simulink model "Realistic_Model"  (R2019a)
settings: Solver=FixedStepAuto  StartTime=0.0  StopTime=200  FixedStep=dt  RelTol=1e-3
values from neighbouring files (symbols this model uses):
  phase_1 = 0    [initMonteCarlo.m]    (also in initRealModel.m; initTrapModel.m)
  phase_2 = 0.005    [initMonteCarlo.m]    (also in initRealModel.m = 0; initTrapModel.m)
  phase_3 = 0    [initRealModel.m]
  phase_4 = 0    [initRealModel.m]
  Q1 = 0.5*60*1000000000    (= 30000000000)    [initMonteCarlo.m]    (also in initRealModel.m = 2000; initTrapModel.m)
  Q2 = 0.5*60*1000000000    (= 30000000000)    [initMonteCarlo.m]    (also in initRealModel.m = 2000; initTrapModel.m)
  Q3 = 2000    [initRealModel.m]
  Q4 = 2000    [initRealModel.m]
  rate_1 = 0.01    [initMonteCarlo.m]    (also in initRealModel.m = 0.3; initTrapModel.m)
  rate_2 = 0.01    [initMonteCarlo.m]    (also in initRealModel.m = 0.3; initTrapModel.m)
  rate_3 = 0.3    [initRealModel.m]
  rate_4 = 0.3    [initRealModel.m]
  seed_1 = 0    [initMonteCarlo.m]    (also in initRealModel.m; initTrapModel.m)
  seed_2 = 1    [initMonteCarlo.m]    (also in initRealModel.m; initTrapModel.m)
  seed_3 = 2    [initRealModel.m]
  seed_4 = 3    [initRealModel.m]
libraries: simulink x8, SinglePipe_lib x7, Junction_Lib x3
settings Model: Creator=martin  LastModifiedBy=martin

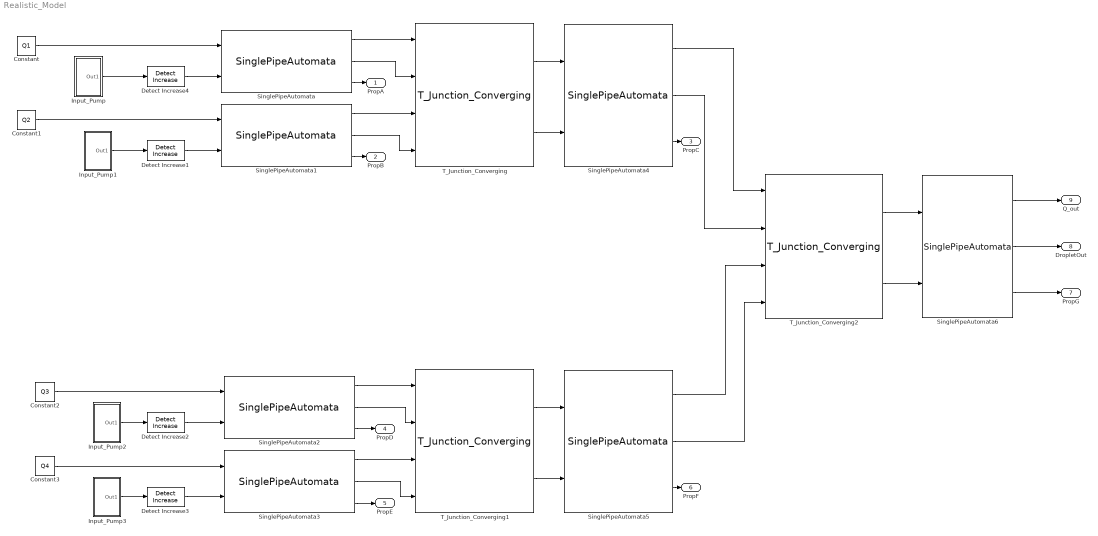
== system Realistic_Model ==
  Constant : Constant  Value=Q1
  Constant1 : Constant  Value=Q2
  Constant2 : Constant  Value=Q3
  Constant3 : Constant  Value=Q4
  Detect Increase{1..4} (4 alike) : simulink/Logic and Bit Operations/Detect Increase  vinit=0  OutDataTypeStr=boolean
  Input_Pump : Subsystem  mask{Period=rate_1, Seed=seed_1, PhaseDelay=phase_1}
      mask prompts: Period "droplet rate"; Seed "Simulink:blkprm_prompts:RandNumInitSeed"; PhaseDelay "Simulink:blkprm_prompts:PulseContPhaseDelay"
      mask TypeOptions Period:
      | Pulse
      | Generator/Period
      mask TypeOptions Seed:
      | Uniform Random
      | Number4/Seed
      mask TypeOptions PhaseDelay:
      | Pulse
      | Generator/PhaseDelay
      mask DialogControl Seed Prompt: Seed:
      mask DialogControl PhaseDelay Prompt: Phase delay (secs):
  Input_Pump1 : Subsystem  mask{Period=rate_2, Seed=seed_2, PhaseDelay=phase_2}
      mask prompts: Period "droplet rate"; Seed "Simulink:blkprm_prompts:RandNumInitSeed"; PhaseDelay "Simulink:blkprm_prompts:PulseContPhaseDelay"
      mask TypeOptions Period:
      | Pulse
      | Generator/Period
      mask TypeOptions Seed:
      | Uniform Random
      | Number4/Seed
      mask TypeOptions PhaseDelay:
      | Pulse
      | Generator/PhaseDelay
      mask DialogControl Seed Prompt: Seed:
      mask DialogControl PhaseDelay Prompt: Phase delay (secs):
  Input_Pump2 : Subsystem  mask{Period=rate_3, Seed=seed_3, PhaseDelay=phase_3}
      mask prompts: Period "droplet rate"; Seed "Simulink:blkprm_prompts:RandNumInitSeed"; PhaseDelay "Simulink:blkprm_prompts:PulseContPhaseDelay"
      mask TypeOptions Period:
      | Pulse
      | Generator/Period
      mask TypeOptions Seed:
      | Uniform Random
      | Number4/Seed
      mask TypeOptions PhaseDelay:
      | Pulse
      | Generator/PhaseDelay
      mask DialogControl Seed Prompt: Seed:
      mask DialogControl PhaseDelay Prompt: Phase delay (secs):
  Input_Pump3 : Subsystem  mask{Period=rate_4, Seed=seed_4, PhaseDelay=phase_4}
      mask prompts: Period "droplet rate"; Seed "Simulink:blkprm_prompts:RandNumInitSeed"; PhaseDelay "Simulink:blkprm_prompts:PulseContPhaseDelay"
      mask TypeOptions Period:
      | Pulse
      | Generator/Period
      mask TypeOptions Seed:
      | Uniform Random
      | Number4/Seed
      mask TypeOptions PhaseDelay:
      | Pulse
      | Generator/PhaseDelay
      mask DialogControl Seed Prompt: Seed:
      mask DialogControl PhaseDelay Prompt: Phase delay (secs):
  SinglePipeAutomata : SinglePipe_lib/SinglePipeAutomata  width=W.A  length=L.A  height=H.A  dt=dt
  SinglePipeAutomata1 : SinglePipe_lib/SinglePipeAutomata  width=W.B  length=L.B  height=H.B  dt=dt
  SinglePipeAutomata2 : SinglePipe_lib/SinglePipeAutomata  width=W.D  length=L.D  height=H.D  dt=dt
  SinglePipeAutomata3 : SinglePipe_lib/SinglePipeAutomata  width=W.E  length=L.E  height=H.E  dt=dt
  SinglePipeAutomata4 : SinglePipe_lib/SinglePipeAutomata  width=W.C  length=L.C  height=H.C  dt=dt
  SinglePipeAutomata5 : SinglePipe_lib/SinglePipeAutomata  width=W.F  length=L.F  height=H.F  dt=dt
  SinglePipeAutomata6 : SinglePipe_lib/SinglePipeAutomata  width=W.G  length=L.G  height=H.G  dt=dt
  T_Junction_Converging : Junction_Lib/T_Junction_Converging  SystemSampleTime=-1
  T_Junction_Converging1 : Junction_Lib/T_Junction_Converging  SystemSampleTime=-1
  T_Junction_Converging2 : Junction_Lib/T_Junction_Converging  SystemSampleTime=-1
  PropA : Outport
  PropB : Outport  Port=2
  PropC : Outport  Port=3
  PropD : Outport  Port=4
  PropE : Outport  Port=5
  PropF : Outport  Port=6
  PropG : Outport  Port=7
  DropletOut : Outport  Port=8
  Q_out : Outport  Port=9
  wires:
  T_Junction_Converging2/1 -> SinglePipeAutomata6/1
  T_Junction_Converging2/2 -> SinglePipeAutomata6/2
  SinglePipeAutomata4/1 -> T_Junction_Converging2/1
  SinglePipeAutomata4/2 -> T_Junction_Converging2/2
  SinglePipeAutomata5/1 -> T_Junction_Converging2/3
  SinglePipeAutomata5/2 -> T_Junction_Converging2/4
  T_Junction_Converging/2 -> SinglePipeAutomata4/2
  T_Junction_Converging/1 -> SinglePipeAutomata4/1
  T_Junction_Converging1/1 -> SinglePipeAutomata5/1
  T_Junction_Converging1/2 -> SinglePipeAutomata5/2
  SinglePipeAutomata2/1 -> T_Junction_Converging1/1
  SinglePipeAutomata2/2 -> T_Junction_Converging1/2
  SinglePipeAutomata3/1 -> T_Junction_Converging1/3
  SinglePipeAutomata3/2 -> T_Junction_Converging1/4
  SinglePipeAutomata/1 -> T_Junction_Converging/1
  SinglePipeAutomata/2 -> T_Junction_Converging/2
  SinglePipeAutomata1/1 -> T_Junction_Converging/3
  SinglePipeAutomata1/2 -> T_Junction_Converging/4
  SinglePipeAutomata/3 -> PropA/1
  SinglePipeAutomata1/3 -> PropB/1
  SinglePipeAutomata4/3 -> PropC/1
  SinglePipeAutomata2/3 -> PropD/1
  SinglePipeAutomata3/3 -> PropE/1
  SinglePipeAutomata5/3 -> PropF/1
  SinglePipeAutomata6/3 -> PropG/1
  SinglePipeAutomata6/2 -> DropletOut/1
  SinglePipeAutomata6/1 -> Q_out/1
  Constant/1 -> SinglePipeAutomata/1
  Constant1/1 -> SinglePipeAutomata1/1
  Constant2/1 -> SinglePipeAutomata2/1
  Constant3/1 -> SinglePipeAutomata3/1
  Detect Increase1/1 -> SinglePipeAutomata1/2
  Detect Increase2/1 -> SinglePipeAutomata2/2
  Detect Increase3/1 -> SinglePipeAutomata3/2
  Detect Increase4/1 -> SinglePipeAutomata/2
  Input_Pump2/1(Out1) -> Detect Increase2/1
  Input_Pump/1(Out1) -> Detect Increase4/1
  Input_Pump1/1(Out1) -> Detect Increase1/1
  Input_Pump3/1(Out1) -> Detect Increase3/1

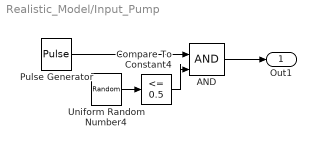
== system Realistic_Model/Input_Pump ==
  AND : Logic  IconShape=distinctive  AllPortsSameDT=off  OutDataTypeStr=boolean
  Compare To Constant4 : simulink/Logic and Bit Operations/Compare To Constant  relop=<=  const=0.5  OutDataTypeStr=boolean
  Pulse Generator : DiscretePulseGenerator  PulseType=Time based  Period=Period  PulseWidth=5  PhaseDelay=PhaseDelay
  Uniform Random Number4 : UniformRandomNumber  Seed=Seed  SampleTime=0.1
  Out1 : Outport
  wires:
  Uniform Random Number4/1 -> Compare To Constant4/1
  Compare To Constant4/1 -> AND/2
  AND/1 -> Out1/1
  Pulse Generator/1 -> AND/1

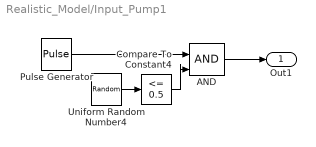
== system Realistic_Model/Input_Pump1 ==
  AND : Logic  IconShape=distinctive  AllPortsSameDT=off  OutDataTypeStr=boolean
  Compare To Constant4 : simulink/Logic and Bit Operations/Compare To Constant  relop=<=  const=0.5  OutDataTypeStr=boolean
  Pulse Generator : DiscretePulseGenerator  PulseType=Time based  Period=Period  PulseWidth=5  PhaseDelay=PhaseDelay
  Uniform Random Number4 : UniformRandomNumber  Seed=Seed  SampleTime=0.1
  Out1 : Outport
  wires:
  Pulse Generator/1 -> AND/1
  AND/1 -> Out1/1
  Compare To Constant4/1 -> AND/2
  Uniform Random Number4/1 -> Compare To Constant4/1

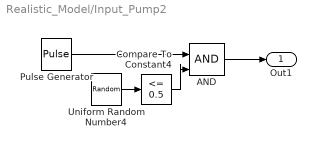
== system Realistic_Model/Input_Pump2 ==
  AND : Logic  IconShape=distinctive  AllPortsSameDT=off  OutDataTypeStr=boolean
  Compare To Constant4 : simulink/Logic and Bit Operations/Compare To Constant  relop=<=  const=0.5  OutDataTypeStr=boolean
  Pulse Generator : DiscretePulseGenerator  PulseType=Time based  Period=Period  PulseWidth=5  PhaseDelay=PhaseDelay
  Uniform Random Number4 : UniformRandomNumber  Seed=Seed  SampleTime=0.1
  Out1 : Outport
  wires:
  Uniform Random Number4/1 -> Compare To Constant4/1
  Compare To Constant4/1 -> AND/2
  AND/1 -> Out1/1
  Pulse Generator/1 -> AND/1

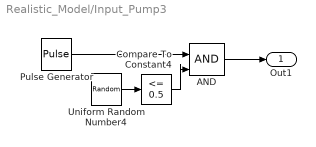
== system Realistic_Model/Input_Pump3 ==
  AND : Logic  IconShape=distinctive  AllPortsSameDT=off  OutDataTypeStr=boolean
  Compare To Constant4 : simulink/Logic and Bit Operations/Compare To Constant  relop=<=  const=0.5  OutDataTypeStr=boolean
  Pulse Generator : DiscretePulseGenerator  PulseType=Time based  Period=Period  PulseWidth=5  PhaseDelay=PhaseDelay
  Uniform Random Number4 : UniformRandomNumber  Seed=Seed  SampleTime=0.1
  Out1 : Outport
  wires:
  Pulse Generator/1 -> AND/1
  AND/1 -> Out1/1
  Compare To Constant4/1 -> AND/2
  Uniform Random Number4/1 -> Compare To Constant4/1
